simulink model "nonlinear_spacecraft_euler"  (R2015b)
settings: Solver=VariableStepAuto  StartTime=0.0  StopTime=10.0  RelTol=1e-3
values from neighbouring files (symbols this model uses):
  B = [zeros(3,3);diag([1/I_x 1/I_y 1/I_z])]    [main_linear_spacecraft_euler.m]
  I_x = 1    [main_linear_spacecraft_euler.m]    (also in main_reaction_nonlinear_v02.m; main_reaction_wheels_detumbling.m; main_reaction_wheels_nonlinear_v01.m; main_reaction_wheels_nonlinear_v03.m)
  I_y = 0.5    [main_linear_spacecraft_euler.m]    (also in main_reaction_nonlinear_v02.m; main_reaction_wheels_detumbling.m; main_reaction_wheels_nonlinear_v01.m; main_reaction_wheels_nonlinear_v03.m)
  I_z = 0.7    [main_linear_spacecraft_euler.m]    (also in main_reaction_nonlinear_v02.m; main_reaction_wheels_detumbling.m; main_reaction_wheels_nonlinear_v01.m; main_reaction_wheels_nonlinear_v03.m)
  x_0 = [phi_0 ... (first row only)    [main_linear_spacecraft_euler.m]    (also in main_reaction_wheels_detumbling.m = [epsilon_0; main_reaction_wheels_nonlinear_v03.m = [epsilon_0)
settings Model: Creator=Krunal's PC  LastModifiedBy=Krunal's PC

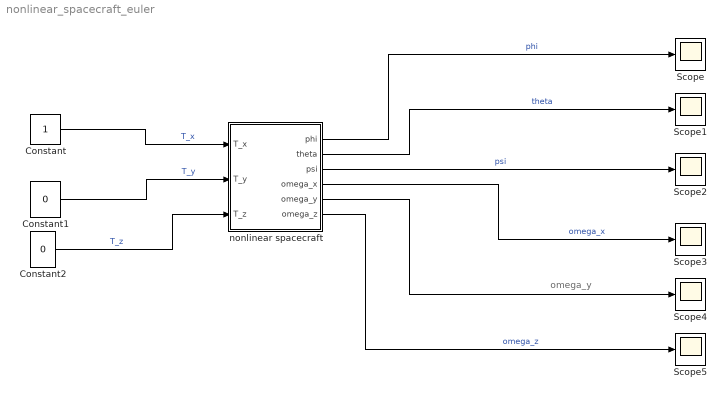
== system nonlinear_spacecraft_euler ==
  note: omega_y
  Constant : Constant
  Constant1 : Constant  Value=0
  Constant2 : Constant  Value=0
  Scope{,1..5} (6 alike) : Scope
  nonlinear spacecraft : Subsystem
  wires:
  Constant/1 -> nonlinear spacecraft/1(T_x)  "T_x"
  Constant1/1 -> nonlinear spacecraft/2(T_y)  "T_y"
  Constant2/1 -> nonlinear spacecraft/3(T_z)  "T_z"
  nonlinear spacecraft/1(phi) -> Scope/1  "phi"
  nonlinear spacecraft/2(theta) -> Scope1/1  "theta"
  nonlinear spacecraft/3(psi) -> Scope2/1  "psi"
  nonlinear spacecraft/4(omega_x) -> Scope3/1  "omega_x"
  nonlinear spacecraft/5(omega_y) -> Scope4/1
  nonlinear spacecraft/6(omega_z) -> Scope5/1  "omega_z"

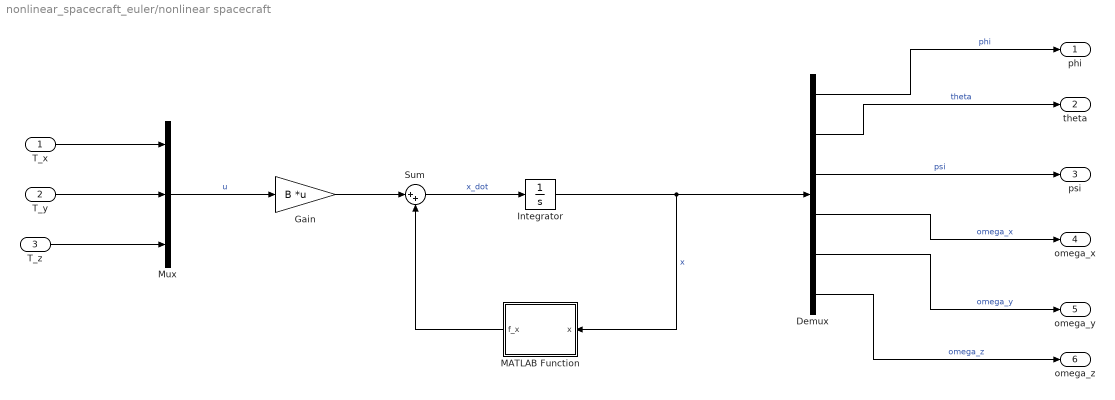
== system nonlinear_spacecraft_euler/nonlinear spacecraft ==
  T_x : Inport
  T_y : Inport  Port=2
  T_z : Inport  Port=3
  Demux : Demux  Outputs=6
  Gain : Gain  Gain=B  Multiplication=Matrix(K*u)
  Integrator : Integrator  InitialCondition=x_0
  MATLAB Function : MATLAB Function  TreatAsAtomicUnit=on
  Mux : Mux  Inputs=3
  Sum : Sum  Inputs=|++
  phi : Outport
  theta : Outport  Port=2
  psi : Outport  Port=3
  omega_x : Outport  Port=4
  omega_y : Outport  Port=5
  omega_z : Outport  Port=6
  wires:
  T_z/1 -> Mux/3
  Integrator/1 -> MATLAB Function/1(x), Demux/1  "x"
  T_y/1 -> Mux/2
  Demux/2 -> theta/1  "theta"
  Demux/6 -> omega_z/1  "omega_z"
  T_x/1 -> Mux/1
  Mux/1 -> Gain/1  "u"
  Demux/5 -> omega_y/1  "omega_y"
  Demux/3 -> psi/1  "psi"
  Demux/1 -> phi/1  "phi"
  Demux/4 -> omega_x/1  "omega_x"
  Gain/1 -> Sum/1
  Sum/1 -> Integrator/1  "x_dot"
  MATLAB Function/1(f_x) -> Sum/2

== matlab function nonlinear_spacecraft_euler/nonlinear spacecraft/MATLAB Function ==
  data: x input; f_x output; I_x parameter; I_y parameter; I_z parameter
function f_x = fcn(x,I_x,I_y,I_z)

phi=x(1);
theta=x(2);
psi=x(3);
omega_x=x(4);
omega_y=x(5);
omega_z=x(6);

f_x=zeros(6,1);

f_x(1,1)= omega_x+sin(phi)*tan(theta)*omega_y+cos(phi)*tan(theta)*omega_z;
f_x(2,1)= cos(phi)*omega_y-sin(phi)*omega_z;
f_x(3,1)=1/cos(theta)*(sin(phi)*omega_y+cos(phi)*omega_z);
f_x(4,1)=(I_y-I_z)/I_x*(omega_y*omega_z);
f_x(5,1)=(I_z-I_x)/I_y*(omega_x*omega_z);
f_x(6,1)=(I_x-I_y)/I_z*(omega_x*omega_y);
